simulink model "MPC_Controller"  (R2019b)
settings: Solver=VariableStepAuto  StartTime=0.0  StopTime=20  RelTol=1e-3
values from neighbouring files (symbols this model uses):
  ts_BallRef = ts_camera    (= 0.033)    [LQG_ball.m]    (also in LQG_plate_ball.m; LQR_ball.m = 0.03; PerformExperiment_CompareModelWithMeasurement.m = ts_camera; Template_PerformExperiment.m = ts_camera)
  UseUserDefinedBallReference = 1    [LQG_ball.m]    (also in LQG_plate_ball.m; LQR_ball.m; PerformExperiment_CompareModelWithMeasurement.m = 0; Template_PerformExperiment.m = 0)
  UseUserDefinedPlateReference = 1    [LQG_ball.m]    (also in LQG_plate_ball.m; LQR_ball.m; PerformExperiment_CompareModelWithMeasurement.m; Template_PerformExperiment.m = 0)
undefined symbols (not defined in the file or in its folder): denc_mi, numc_mi
libraries: mpclib x1
settings Model: Creator=Duin home  LastModifiedBy=123
settings ModelReferenceCC: ModelReferenceNumInstancesAllowed=Single

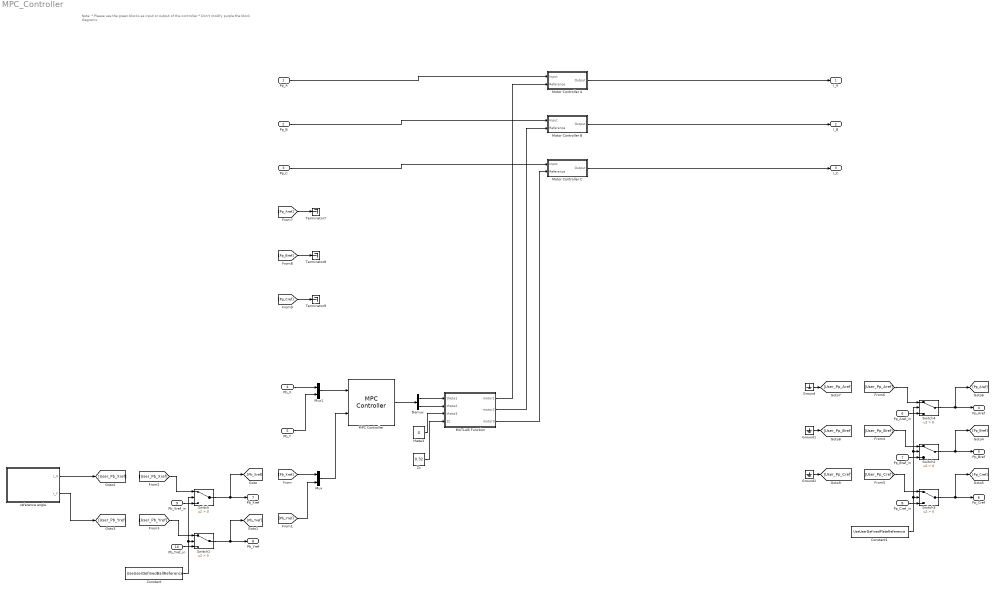
== system MPC_Controller ==
  note: Note:
      | * Please use the green blocks as input or output of the controller
      | * Don't modify purple the block diagrams.
  Pp_A : Inport
  Pp_B : Inport  Port=2
  Pp_C : Inport  Port=3
  Pb_X : Inport  Port=4
  Pb_Y : Inport  Port=5
  Pp_Aref_in : Inport  Port=6
  Pp_Bref_in : Inport  Port=7
  Pp_Cref_in : Inport  Port=8
  Pb_Xref_in : Inport  Port=9
  Pb_Yref_in : Inport  Port=10
  Constant : Constant  Value=UseUserDefinedBallReference
  Constant1 : Constant  Value=UseUserDefinedPlateReference
  Demux : Demux  Outputs=2
  Ground : Ground
  Ground1 : Ground
  Ground2 : Ground
  MATLAB Function : MATLAB Function  TreatAsAtomicUnit=on
  MPC Controller : mpclib/MPC Controller  SCDEnableBlockLinearizationSpecification=on  mpcobj=mpc_controller  is_multiple=0  enable_value=0  return_u0=off  updateMPCinCallerWorkspace=on  md_inport=off  mv_inport=off  uref_inport=off  return_cost=off  return_mvseq=off  return_qpstatus=off  return_xseq=off  return_state=off  return_ovseq=off  state_inport=off  umin_inport=off  umax_inport=off  ymin_inport=off  ymax_inport=off  cc_inport=off  ywt_inport=off  uwt_inport=off  duwt_inport=off  rhoeps_inport=off  pm_inport=off  MaximumP=10  HorizonChoice=FixedHorizon  n_ts=0.04  n_p=5  n_mv=2  n_md=0  n_ud=0  n_mo=2  n_uo=0  BlockDataType=double  SampleTimeInherited=off  switch_inport=off
  Motor Controller A : Subsystem
  Motor Controller B : Subsystem
  Motor Controller C : Subsystem
  Mux : Mux  Inputs=2
  Mux1 : Mux  Inputs=2
  Switch{,1..4} (5 alike) : Switch  Criteria=u2 > Threshold
  Terminator7 : Terminator
  Terminator8 : Terminator
  Terminator9 : Terminator
  Zc : Constant  Value=0.32
  reference angle : Subsystem
  theta3 : Constant  Value=0
  I_A : Outport
  I_B : Outport  Port=2
  I_C : Outport  Port=3
  Pp_Aref : Outport  Port=4
  Pp_Bref : Outport  Port=5
  Pp_Cref : Outport  Port=6
  Pb_Xref : Outport  Port=7
  Pb_Yref : Outport  Port=8
  wires:
  Pp_A/1 -> Motor Controller A/1(Input)
  Pp_B/1 -> Motor Controller B/1(Input)
  Pp_C/1 -> Motor Controller C/1(Input)
  Motor Controller C/1(Output) -> I_C/1
  Motor Controller B/1(Output) -> I_B/1
  Motor Controller A/1(Output) -> I_A/1
  MATLAB Function/3(motor3) -> Motor Controller C/2(Reference)
  MATLAB Function/2(motor2) -> Motor Controller B/2(Reference)
  MATLAB Function/1(motor1) -> Motor Controller A/2(Reference)
  Pb_Xref_in/1 -> Switch/3
  Pb_Yref_in/1 -> Switch1/3
  Switch1/1 -> [Pb_Yref], Pb_Yref/1
  Switch/1 -> [Pb_Xref], Pb_Xref/1
  [User_Pb_Xref] -> Switch/1
  [User_Pb_Yref] -> Switch1/1
  Constant/1 -> Switch/2, Switch1/2
  reference angle/1(r_X) -> [User_Pb_Xref]
  reference angle/2(r_Y) -> [User_Pb_Yref]
  [Pb_Yref] -> Mux/2
  [Pb_Xref] -> Mux/1
  Pp_Bref_in/1 -> Switch2/3
  [User_Pp_Bref] -> Switch2/1
  Switch3/1 -> [Pp_Cref], Pp_Cref/1
  Switch2/1 -> [Pp_Bref], Pp_Bref/1
  Pp_Cref_in/1 -> Switch3/3
  Constant1/1 -> Switch4/2, Switch2/2, Switch3/2
  [User_Pp_Cref] -> Switch3/1
  [User_Pp_Aref] -> Switch4/1
  Pp_Aref_in/1 -> Switch4/3
  Switch4/1 -> [Pp_Aref], Pp_Aref/1
  [Pp_Bref] -> Terminator8/1
  [Pp_Aref] -> Terminator7/1
  [Pp_Cref] -> Terminator9/1
  Mux/1 -> MPC Controller/2
  Pb_X/1 -> Mux1/1
  Pb_Y/1 -> Mux1/2
  Mux1/1 -> MPC Controller/1
  MPC Controller/1 -> Demux/1
  Demux/1 -> MATLAB Function/1(theta1)
  Demux/2 -> MATLAB Function/2(theta2)
  theta3/1 -> MATLAB Function/3(theta3)
  Zc/1 -> MATLAB Function/4(Zc)
  Ground/1 -> [User_Pp_Aref]
  Ground1/1 -> [User_Pp_Bref]
  Ground2/1 -> [User_Pp_Cref]

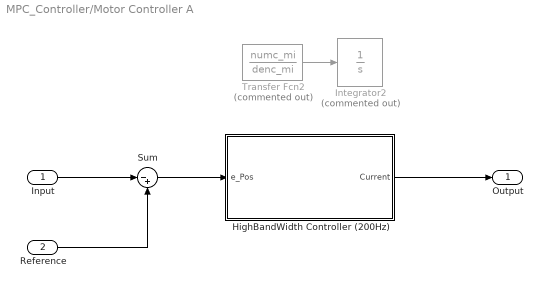
== system MPC_Controller/Motor Controller A ==
  Input : Inport
  Reference : Inport  Port=2
  HighBandWidth Controller (200Hz) : Subsystem
  Integrator2 : Integrator  Commented=on  LimitOutput=on  UpperSaturationLimit=3  LowerSaturationLimit=-3
  Sum : Sum  Inputs=|-+
  Transfer Fcn2 : TransferFcn  Commented=on  Numerator=numc_mi  Denominator=denc_mi
  Output : Outport
  wires:
  Input/1 -> Sum/1
  Reference/1 -> Sum/2
  HighBandWidth Controller (200Hz)/1(Current) -> Output/1
  Sum/1 -> HighBandWidth Controller (200Hz)/1(e_Pos)
  Transfer Fcn2/1 -> Integrator2/1

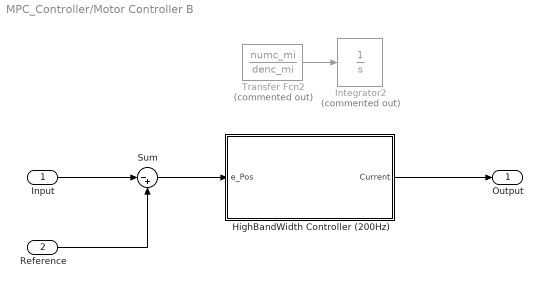
== system MPC_Controller/Motor Controller B ==
  Input : Inport
  Reference : Inport  Port=2
  HighBandWidth Controller (200Hz) : Subsystem
  Integrator2 : Integrator  Commented=on  LimitOutput=on  UpperSaturationLimit=3  LowerSaturationLimit=-3
  Sum : Sum  Inputs=|-+
  Transfer Fcn2 : TransferFcn  Commented=on  Numerator=numc_mi  Denominator=denc_mi
  Output : Outport
  wires:
  HighBandWidth Controller (200Hz)/1(Current) -> Output/1
  Sum/1 -> HighBandWidth Controller (200Hz)/1(e_Pos)
  Input/1 -> Sum/1
  Reference/1 -> Sum/2
  Transfer Fcn2/1 -> Integrator2/1

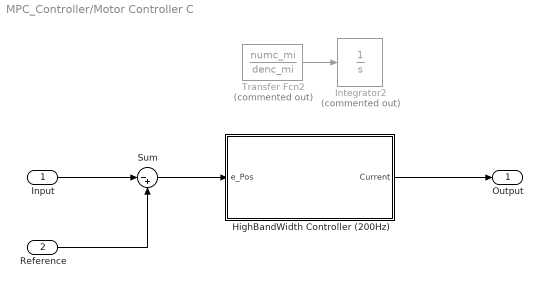
== system MPC_Controller/Motor Controller C ==
  Input : Inport
  Reference : Inport  Port=2
  HighBandWidth Controller (200Hz) : Subsystem
  Integrator2 : Integrator  Commented=on  LimitOutput=on  UpperSaturationLimit=3  LowerSaturationLimit=-3
  Sum : Sum  Inputs=|-+
  Transfer Fcn2 : TransferFcn  Commented=on  Numerator=numc_mi  Denominator=denc_mi
  Output : Outport
  wires:
  HighBandWidth Controller (200Hz)/1(Current) -> Output/1
  Sum/1 -> HighBandWidth Controller (200Hz)/1(e_Pos)
  Input/1 -> Sum/1
  Reference/1 -> Sum/2
  Transfer Fcn2/1 -> Integrator2/1

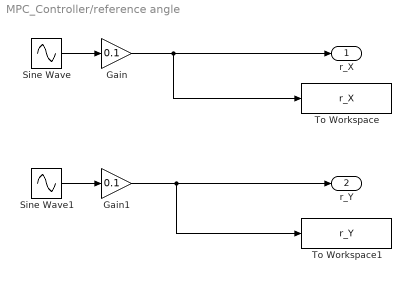
== system MPC_Controller/reference angle ==
  Gain : Gain  Gain=0.1
  Gain1 : Gain  Gain=0.1
  Sine Wave : Sin  Frequency=0.5  SampleTime=ts_BallRef
  Sine Wave1 : Sin  Frequency=0.5  Phase=pi/2  SampleTime=ts_BallRef
  To Workspace : ToWorkspace  VariableName=r_X  SampleTime=-1
  To Workspace1 : ToWorkspace  VariableName=r_Y  SampleTime=-1
  r_X : Outport
  r_Y : Outport  Port=2
  wires:
  Sine Wave/1 -> Gain/1
  Sine Wave1/1 -> Gain1/1
  Gain/1 -> To Workspace/1, r_X/1
  Gain1/1 -> r_Y/1, To Workspace1/1

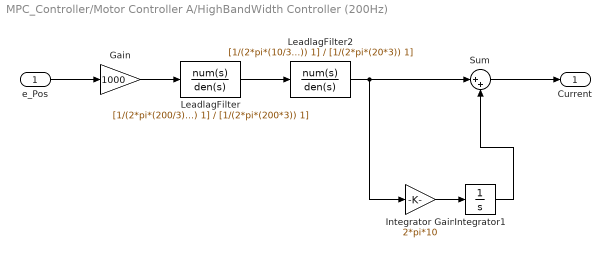
== system MPC_Controller/Motor Controller A/HighBandWidth Controller (200Hz) ==
  e_Pos : Inport
  Gain : Gain  Gain=1000
  Integrator Gain : Gain  Gain=2*pi*10
  Integrator1 : Integrator  LimitOutput=on  UpperSaturationLimit=3  LowerSaturationLimit=-3
  LeadlagFilter : TransferFcn  Numerator=[1/(2*pi*(200/3)) 1]  Denominator=[1/(2*pi*(200*3)) 1]
  LeadlagFilter2 : TransferFcn  Numerator=[1/(2*pi*(10/3)) 1]  Denominator=[1/(2*pi*(20*3)) 1]
  Sum : Sum  Inputs=|++
  Current : Outport
  wires:
  Gain/1 -> LeadlagFilter/1
  e_Pos/1 -> Gain/1
  Integrator Gain/1 -> Integrator1/1
  Sum/1 -> Current/1
  Integrator1/1 -> Sum/2
  LeadlagFilter/1 -> LeadlagFilter2/1
  LeadlagFilter2/1 -> Integrator Gain/1, Sum/1

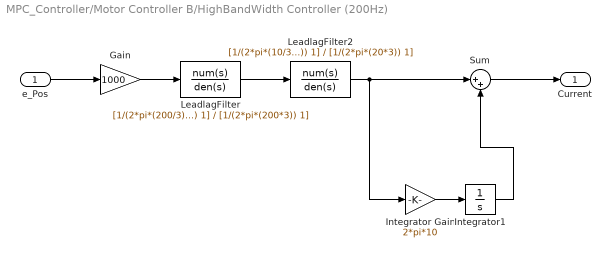
== system MPC_Controller/Motor Controller B/HighBandWidth Controller (200Hz) ==
  e_Pos : Inport
  Gain : Gain  Gain=1000
  Integrator Gain : Gain  Gain=2*pi*10
  Integrator1 : Integrator  LimitOutput=on  UpperSaturationLimit=3  LowerSaturationLimit=-3
  LeadlagFilter : TransferFcn  Numerator=[1/(2*pi*(200/3)) 1]  Denominator=[1/(2*pi*(200*3)) 1]
  LeadlagFilter2 : TransferFcn  Numerator=[1/(2*pi*(10/3)) 1]  Denominator=[1/(2*pi*(20*3)) 1]
  Sum : Sum  Inputs=|++
  Current : Outport
  wires:
  Gain/1 -> LeadlagFilter/1
  e_Pos/1 -> Gain/1
  Integrator Gain/1 -> Integrator1/1
  Sum/1 -> Current/1
  Integrator1/1 -> Sum/2
  LeadlagFilter/1 -> LeadlagFilter2/1
  LeadlagFilter2/1 -> Integrator Gain/1, Sum/1

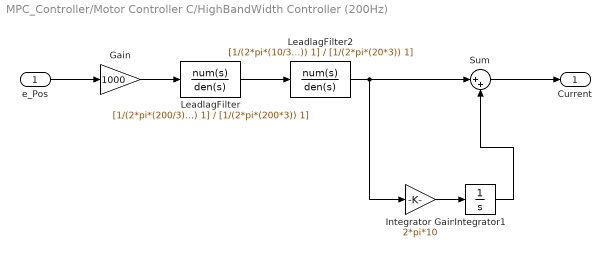
== system MPC_Controller/Motor Controller C/HighBandWidth Controller (200Hz) ==
  e_Pos : Inport
  Gain : Gain  Gain=1000
  Integrator Gain : Gain  Gain=2*pi*10
  Integrator1 : Integrator  LimitOutput=on  UpperSaturationLimit=3  LowerSaturationLimit=-3
  LeadlagFilter : TransferFcn  Numerator=[1/(2*pi*(200/3)) 1]  Denominator=[1/(2*pi*(200*3)) 1]
  LeadlagFilter2 : TransferFcn  Numerator=[1/(2*pi*(10/3)) 1]  Denominator=[1/(2*pi*(20*3)) 1]
  Sum : Sum  Inputs=|++
  Current : Outport
  wires:
  Gain/1 -> LeadlagFilter/1
  e_Pos/1 -> Gain/1
  Integrator Gain/1 -> Integrator1/1
  Sum/1 -> Current/1
  Integrator1/1 -> Sum/2
  LeadlagFilter/1 -> LeadlagFilter2/1
  LeadlagFilter2/1 -> Integrator Gain/1, Sum/1

== matlab function MPC_Controller/MATLAB Function ==
  data: theta1 input; motor1 output; theta2 input; theta3 input; Zc input; motor2 output; motor3 output
function [motor1, motor2, motor3] = anglesToMotors(theta1,theta2,theta3,Zc)

%% Define parameters
r = 0.17;
r0B1 = [r; 0; 0];      
r0B2 = [-0.5*r; (sqrt(3)/2)*r; 0];
r0B3 = [-0.5*r; -(sqrt(3)/2)*r; 0];
r0B = [r0B1 r0B2 r0B3];
%r1C1 = r0B1; r1C2 = r0B2; r1C3 = r0B3;
r1C = r0B;
r0Oc = [0;0;Zc];

% Find cos and sin to accelerate calculations
C1 = cos(theta1);S1 = sin(theta1);C2 = cos(theta2);S2 = sin(theta2);C3 = cos(theta3);S3 = sin(theta3);

% Rotation matrices
RotZ = [C3 S3 0; -S3 C3 0; 0 0 1];
RotY = [C2 0 -S2; 0 1 0; S2 0 C2];
RotX = [1 0 0; 0 C1 S1; 0 -S1 C1];

A10 = RotX*RotY*RotZ; A01 = A10';

% Find rCiBi (Vectors representing the motors)
rCiBi = zeros(3,3);
for i=1:3
    rCiBi(:,i) = r0Oc + A01*r1C(:,i) - r0B(:,i);
end

% Outputs to motor are the lengths of the vectors
motor1 = norm(rCiBi(:,1));
motor2 = norm(rCiBi(:,2));
motor3 = norm(rCiBi(:,3));
end
